simulink model "Compressing"  (R2016a)
settings: Solver=VariableStepAuto  StartTime=0.0  StopTime=0  RelTol=1e-3
values from neighbouring files (symbols this model uses):
  bits = 16    [Cepstrum_Compression.m]    (also in Cepstrum_Compression_Simulink.m = 20)
  col = N    [Cepstrum_Compression.m]    (also in Cepstrum_Compression_Simulink.m)
  N = data(1,end)    [Cepstrum_Compression.m]    (also in Cepstrum_Compression_Simulink.m)
  row = ceil(length(x)/N)    [Cepstrum_Compression.m]    (also in Cepstrum_Compression_Simulink.m)
  x = zeros(1,row*N)    [Cepstrum_Compression.m]    (also in Cepstrum_Compression_Simulink.m = x')
libraries: dspmtrx3 x3, visionstatistics x1, dspsigops x1
settings Model: Creator=HP  LastModifiedBy=HP

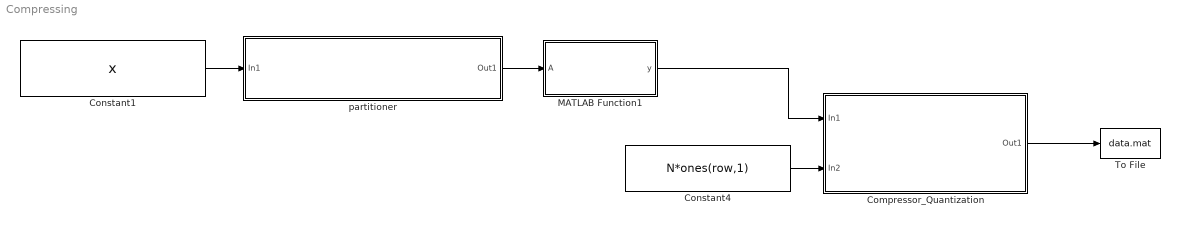
== system Compressing ==
  Compressor_Quantization : Subsystem
  Constant1 : Constant  Value=x
  Constant4 : Constant  Value=N*ones(row,1)
  MATLAB Function1 : MATLAB Function  TreatAsAtomicUnit=on
  To File : ToFile  Filename=data.mat  MatrixName=data  SaveFormat=Timeseries
  partitioner : Subsystem
  wires:
  Constant1/1 -> partitioner/1(In1)
  partitioner/1(Out1) -> MATLAB Function1/1(A)
  MATLAB Function1/1(y) -> Compressor_Quantization/1(In1)
  Constant4/1 -> Compressor_Quantization/2(In2)
  Compressor_Quantization/1(Out1) -> To File/1

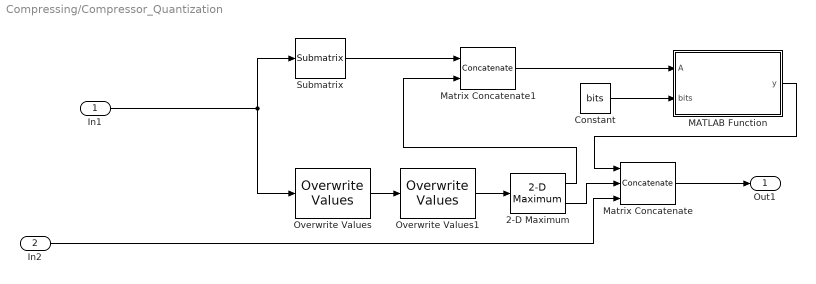
== system Compressing/Compressor_Quantization ==
  In1 : Inport
  In2 : Inport  Port=2
  2-D Maximum : visionstatistics/2-D Maximum  fcn=Value and Index  reset=None  indexBase=One  operateOver=Each row  Dimension=1  colComp=on  operation=maximum  roiEnable=off  roiType=Rectangles  roiPortion=Entire ROI  roiOutput=Individual statistics for each ROI  roiFlag=off  accumDataTypeStr=Inherit: Same as product output  accumLastDataTypeStr=Inherit: Same as product output  roundingMode=Floor  overflowMode=off
  Constant : Constant  Value=bits
  MATLAB Function : MATLAB Function  TreatAsAtomicUnit=on
  Matrix Concatenate : Concatenate  NumInputs=3  Mode=Multidimensional array  ConcatenateDimension=2
  Matrix Concatenate1 : Concatenate  Mode=Multidimensional array  ConcatenateDimension=2
  Overwrite Values : dspmtrx3/Overwrite Values  OverWriteDiag=Submatrix  valFrom2ndIP=Specify via dialog  ConstValue=0  RowSpan=Range of rows  RowStartMode=First  RowStartIndex=1  RowEndMode=Last  RowEndIndex=1  ColSpan=Range of columns  ColStartMode=First  ColStartIndex=1  ColEndMode=Index  ColEndIndex=mem  DiagSpan=Range of elements  DiagStartMode=Index  DiagStartIndex=2  DiagEndMode=Index  DiagEndIndex=4
  Overwrite Values1 : dspmtrx3/Overwrite Values  OverWriteDiag=Submatrix  valFrom2ndIP=Specify via dialog  ConstValue=0  RowSpan=Range of rows  RowStartMode=First  RowStartIndex=1  RowEndMode=Last  RowEndIndex=1  ColSpan=Range of columns  ColStartMode=Index  ColStartIndex=N/2  ColEndMode=Last  ColEndIndex=mem  DiagSpan=Range of elements  DiagStartMode=Index  DiagStartIndex=2  DiagEndMode=Index  DiagEndIndex=4
  Submatrix : dspmtrx3/Submatrix  RowSpan=Range of rows  RowStartMode=First  RowStartIndex=1  RowEndMode=Last  RowEndIndex=1  ColSpan=Range of columns  ColStartMode=First  ColStartIndex=1  ColEndMode=Index  ColEndIndex=mem
  Out1 : Outport
  wires:
  In1/1 -> Overwrite Values/1, Submatrix/1
  In2/1 -> Matrix Concatenate/3
  Matrix Concatenate/1 -> Out1/1
  Overwrite Values/1 -> Overwrite Values1/1
  Submatrix/1 -> Matrix Concatenate1/1
  Overwrite Values1/1 -> 2-D Maximum/1
  2-D Maximum/2 -> Matrix Concatenate/2
  Matrix Concatenate1/1 -> MATLAB Function/1(A)
  2-D Maximum/1 -> Matrix Concatenate1/2
  MATLAB Function/1(y) -> Matrix Concatenate/1
  Constant/1 -> MATLAB Function/2(bits)

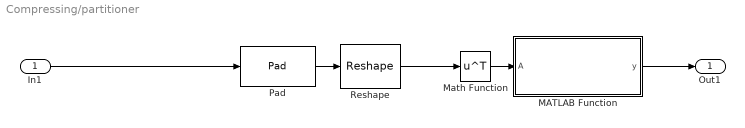
== system Compressing/partitioner ==
  In1 : Inport
  MATLAB Function : MATLAB Function  TreatAsAtomicUnit=on
  Math Function : Math  Operator=transpose  SaturateOnIntegerOverflow=on
  Pad : dspsigops/Pad  padAlong=Rows  dimsToPad=1  valSrc=Specify via dialog  padVal=0  spec=Output size  padNumOutRowsSpecMethod=User-specified  numOutRows=1  padNumOutColsSpecMethod=User-specified  numOutCols=col*row  isVarDimsMode=off  padBeginning=0  padEnd=0  outSizeMode=User-specified  outSize=1  padSigAt=End  trunc_flag=None  roundingMode=Floor  overflowMode=off  truncOrWrapMode=Truncate  wrap_flag=None
  Reshape : Reshape  OutputDimensionality=Customize  OutputDimensions=[col,row]
  Out1 : Outport
  wires:
  MATLAB Function/1(y) -> Out1/1
  Pad/1 -> Reshape/1
  In1/1 -> Pad/1
  Reshape/1 -> Math Function/1
  Math Function/1 -> MATLAB Function/1(A)

== matlab function Compressing/MATLAB Function1 ==
  data: A input; y output
function y = real_cepstrum(A)
[row,col] = size(A);
coder.extrinsic('rceps')
y = zeros(row,col);
for i = 1:row
   A(i,:) = rceps(A(i,:)); 
end
y = A;

== matlab function Compressing/partitioner/MATLAB Function ==
  data: A input; y output
function y = window_hamming(A)
[row,col] = size(A);
coder.extrinsic('hamming')
y = zeros(row,col);
w = zeros(1,col);
w = hamming(col)';
for i = 1:row
   A(i,:) = A(i,:).*w; 
end
y = A;

== matlab function Compressing/Compressor_Quantization/MATLAB Function ==
  data: A input; y output; bits input
function y = Quantization(A,bits)
%#codegen
[row,col] = size(A);
y = zeros(row,col);
B = bits -1;
Xm = max(max(abs(A)));
delta = Xm/2^B;
A = delta.*round(A./delta);

y = A;
